simulink model "AA6"  (Simulink 10.3)
settings: Solver=VariableStepAuto  StartTime=0.0  StopTime=100  RelTol=1e-3
settings Model: Creator=jhaid  LastModifiedBy=jhaid
settings DataIOCC: SaveFormat=Dataset  SignalLoggingSaveFormat=Dataset  ReturnWorkspaceOutputs=on
settings OptimizationCC: ExpressionDepthLimit=128  LifeSpan=auto
settings DebuggingCC: UnderspecifiedInitializationDetection=Simplified  MergeDetectMultiDrivingBlocksExec=error  FcnCallInpInsideContextMsg=error  StateNameClashWarn=none  SFUnexpectedBacktrackingDiag=error  SFNoUnconditionalDefaultTransitionDiag=error  SFExecutionAtInitializationDiag=warning  SFMachineParentedDataDiag=error
settings HardwareCC: ProdBitPerPointer=64  ProdBitPerSizeT=64  ProdBitPerPtrDiffT=64  ProdLargestAtomicFloat=Float  ProdIntDivRoundTo=Zero  ProdEndianess=LittleEndian  ProdWordSize=64  ProdHWDeviceType=Intel->x86-64 (Windows64)
settings ModelReferenceCC: PropagateSignalLabelsOutOfModel=on
settings SFSimCC: SimUseLocalCustomCode=on
settings RTWCC: RTWUseLocalCustomCode=on
settings GRTTargetCC: TargetLangStandard=C99 (ISO)  CombineOutputUpdateFcns=on  GRTInterface=off
settings ConfigComp: CovMetricSettings=dwe  CovSaveCumulativeToWorkspaceVar=off  CovSaveSingleToWorkspaceVar=off  CovExternalEMLEnable=on

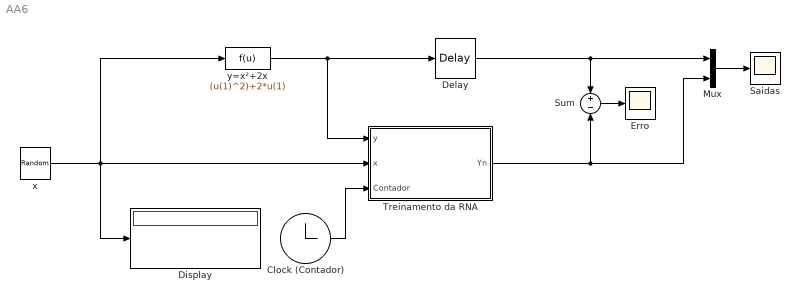
== system AA6 ==
  Clock (Contador) : Clock
  Delay : TransportDelay
  Display : Display
  Erro : Scope
  Mux : Mux  Inputs=2
  Saidas : Scope
  Sum : Sum  Inputs=+|-
  Treinamento da RNA : Subsystem
  x : UniformRandomNumber  Minimum=0  SampleTime=1
  y=x²+2x : Fcn  Expr=(u(1)^2)+2*u(1)
  wires:
  y=x²+2x/1 -> Treinamento da RNA/1(y), Delay/1
  Sum/1 -> Erro/1
  Mux/1 -> Saidas/1
  x/1 -> y=x²+2x/1, Display/1, Treinamento da RNA/2(x)
  Clock (Contador)/1 -> Treinamento da RNA/3(Contador)
  Treinamento da RNA/1("Yn ") -> Mux/2, Sum/2
  Delay/1 -> Sum/1, Mux/1

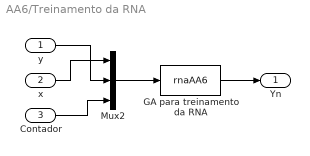
== system AA6/Treinamento da RNA ==
  y : Inport
  x : Inport  Port=2
  Contador : Inport  Port=3
  GA para treinamento da RNA : S-Function  FunctionName=rnaAA6  SFunctionDeploymentMode=off  EnableBusSupport=off
  Mux2 : Mux  Inputs=3
  "Yn " : Outport
  wires:
  Mux2/1 -> GA para treinamento da RNA/1
  y/1 -> Mux2/2
  x/1 -> Mux2/1
  GA para treinamento da RNA/1 -> "Yn "/1
  Contador/1 -> Mux2/3
